simulink model "sldemo_tc"  (R2024a)
settings: Solver=ode3  StartTime=0.0  StopTime=10.0  FixedStep=0.005  RelTol=1e-3
StartFcn:
  | set_param('sldemo_tc/Scope','Open','on')
model workspace (MAT data in the model file):
  TypeS_E_Volts = [-0.000236 -0.000232 -0.000228 -0.000224 -0.000219 -0.000215 -0.000211 -0.000207 -0.000203 -0.000199 -0.000194 -0.00019 ... (1816 elements, 1816x1)]
  TypeS_T_degC = [-50 -49 -48 -47 -46 -45 -44 -43 -42 -41 -40 -39 ... (1816 elements, 1816x1)]
  TypeS_bits_bp = [0 50 100 150 200 250 300 350 400 450 500 550 ... (83 elements, 83x1)]
  TypeS_tdegc_interp = [-50 -1.05395507812 38.4789352417 73.4326858521 105.529296875 135.797668457 164.757202148 192.63710022 219.712234497 246.231826782 272.095336914 297.6043396 ... (83 elements, 83x1)]
  TypeS_tdegc_vs_bits = [-50 -48.8466186523 -47.6932373047 -46.6318855286 -45.6364746094 -44.4830932617 -43.3297119141 -42.1763305664 -41.0229492188 -40.0956535339 -38.9661865234 -37.8502426147 ... (4096 elements, 4096x1)]
  e_vs_counts = [-0.236 -0.231386474609 -0.226772949219 -0.222159423828 -0.217545898437 -0.212932373047 -0.208318847656 -0.203705322266 -0.199091796875 -0.194478271484 -0.189864746094 -0.185251220703 ... (4096 elements, 4096x1)]
libraries: simulink_extras x1
(part 2 of 2)

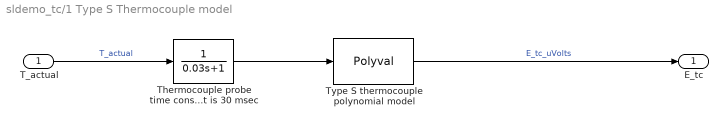
== system sldemo_tc/1 Type S Thermocouple model ==
  T_actual : Inport  Unit=degC
  Thermocouple probe time constant is 30 msec : TransferFcn  Denominator=[0.03 1]
  Type S thermocouple polynomial model : Polyval  Description=|  Coefs=[ +2.71443176145e-021, -1.25068871393e-017, +2.55744251786e-014, -3.31465196389e-011, +3.22028823036e-008, -2.32477968689e-005, +1.25934289740e-002, +5.40313308631e+000, +0.00000000000e+000 ]
      | 0 deg C ice reference         
      |       microVolts = f(Temperature degC)   
      | (Segment 1) input range: -50 to 1063 degC
      settings: AttributesFormatString=%<Description>
  E_tc : Outport  Unit=uV  VectorParamsAs1DForOutWhenUnconnected=off
  wires:
  Thermocouple probe time constant is 30 msec/1 -> Type S thermocouple polynomial model/1
  T_actual/1 -> Thermocouple probe time constant is 30 msec/1  "T_actual"
  Type S thermocouple polynomial model/1 -> E_tc/1  "E_tc_uVolts"

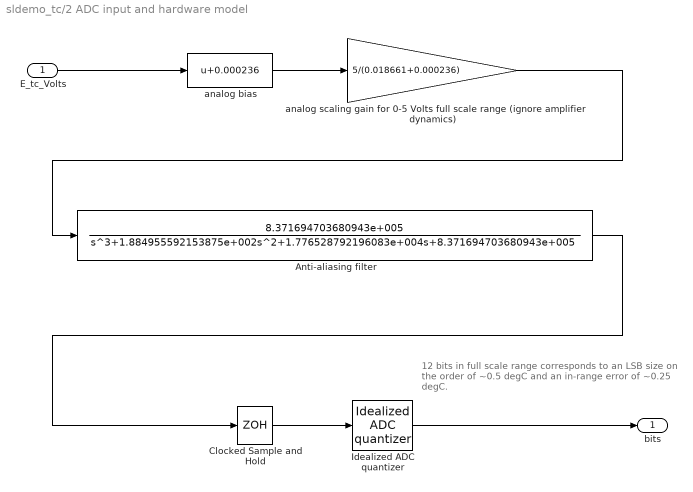
== system sldemo_tc/2 ADC input and hardware model ==
  note: 12 bits in full scale range corresponds to
      | an LSB size on the order of ~0.5 degC and
      | an in-range error of ~0.25 degC.
  E_tc_Volts : Inport  Unit=V
  Anti-aliasing filter : TransferFcn  Description=|  Numerator=8.371694703680943e+005  Denominator=[ 1, 1.884955592153875e+002, 1.776528792196083e+004, 8.371694703680943e+005 ]
      | Designed using Signal Processing Toolbox command:
      | >> [num,den] = butter(3,15*2*pi,'low','s')
      settings: AttributesFormatString=%<Description>
  Clocked Sample and Hold : ZeroOrderHold  SampleTime=0.020
      settings: AttributesFormatString=(%<SampleTime> sec)
  Idealized ADC quantizer : simulink_extras/Additional Discrete/Idealized ADC quantizer  NumberOfConverterBits=12  Vmin=0  Vmax=5  OutputDataType=uint16  OutputNegativeValues=off
      settings: SourceProductName=Simulink
  analog bias : Bias  Bias=0.000236  SaturateOnIntegerOverflow=off
  analog scaling gain for 0-5 Volts full scale range (ignore amplifier dynamics) : Gain  Gain=5/(0.018661+0.000236)
  bits : Outport  Unit=count  VectorParamsAs1DForOutWhenUnconnected=off
  wires:
  analog scaling gain for 0-5 Volts full scale range (ignore amplifier dynamics)/1 -> Anti-aliasing filter/1
  E_tc_Volts/1 -> analog bias/1
  Clocked Sample and Hold/1 -> Idealized ADC quantizer/1
  Idealized ADC quantizer/1 -> bits/1
  analog bias/1 -> analog scaling gain for 0-5 Volts full scale range (ignore amplifier dynamics)/1
  Anti-aliasing filter/1 -> Clocked Sample and Hold/1

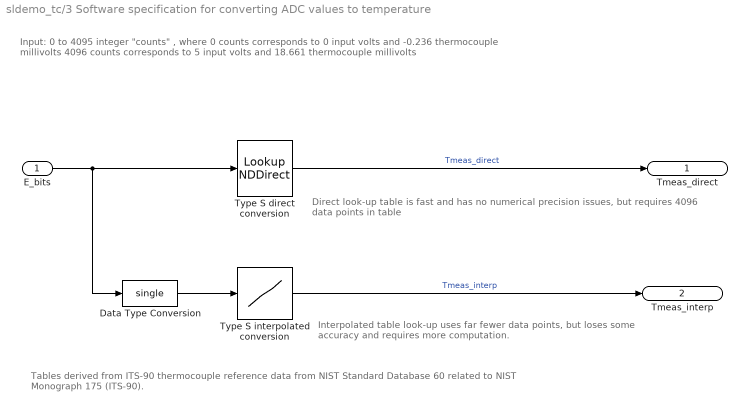
== system sldemo_tc/3 Software specification for converting ADC values to temperature ==
  note: Input: 0 to 4095 integer "counts" , where
      |             0        counts corresponds to 0 input volts and -0.236 thermocouple millivolts
      |             4096 counts corresponds to 5 input volts and 18.661 thermocouple millivolts
  note: Tables derived from ITS-90 thermocouple reference data
      | from NIST Standard Database 60 related to NIST Monograph 175 (ITS-90).
  note: Direct look-up table is fast and has no numerical precision issues,
      | but requires 4096 data points in table
  note: Interpolated table look-up uses far fewer data points,
      | but loses some accuracy and requires more computation.
  E_bits : Inport  OutDataTypeStr=uint16  Unit=count
  Data Type Conversion : DataTypeConversion  OutDataTypeStr=single  SaturateOnIntegerOverflow=off  RndMeth=Floor
  Type S direct conversion : LookupNDDirect  NumberOfTableDimensions=1  Table=TypeS_tdegc_vs_bits
      settings: AttributesFormatString=(%<mxTable>)
  Type S interpolated conversion : Lookup_n-D  NumberOfTableDimensions=1  BreakpointsForDimension1=TypeS_bits_bp  IndexSearchMethod=Linear search  BeginIndexSearchUsingPreviousIndexResult=on  Table=TypeS_tdegc_interp  ExtrapMethod=Clip  DiagnosticForOutOfRangeInput=Warning  InternalRulePriority=Speed  RndMeth=Simplest
      settings: AttributesFormatString=(%<tableData>)
  Tmeas_direct : Outport  Unit=degC  VectorParamsAs1DForOutWhenUnconnected=off
  Tmeas_interp : Outport  Port=2  Unit=degC  VectorParamsAs1DForOutWhenUnconnected=off
  wires:
  E_bits/1 -> Type S direct conversion/1, Data Type Conversion/1
  Type S direct conversion/1 -> Tmeas_direct/1  "Tmeas_direct"
  Data Type Conversion/1 -> Type S interpolated conversion/1
  Type S interpolated conversion/1 -> Tmeas_interp/1  "Tmeas_interp"

== system sldemo_tc/More Info ==

== system sldemo_tc/z: jump to ADC example ==
  note: This block intentionally has no contents.

== system sldemo_tc/z: jump to prebuilt models ==
  note: This block intentionally has no contents.

== system sldemo_tc/z: jump to table data file ==
  note: This block intentionally has no contents.
